simulink model "TFlex_PID"  (R2018a)
settings: Solver=FixedStepDiscrete  StartTime=0.0  StopTime=t_end  FixedStep=ts  RelTol=1e-3
PreLoadFcn:
  | Ts = 0.001;
InitFcn:
  | Ts = 0.001;
values from neighbouring files (symbols this model uses):
  a0 = omega_n^3    (= 31006276.6803)    [Tflex_PID_init.m]
  a1 = 3*omega_n^2    (= 296088.132033)    [Tflex_PID_init.m]
  a2 = 3*omega_n    (= 942.477796077)    [Tflex_PID_init.m]
  b = ones(2*D,Q)*0.001    [Tflex_PID_init.m]
  D = 21    [Tflex_PID_init.m]
  I_limit_max = 500    [Tflex_PID_init.m]
  I_limit_min = -500    [Tflex_PID_init.m]
  Kd = kp*(tau_z-tau_p*(1+(tau_z+tau_p)/tau_i))    [Tflex_PID_init.m]
  Ki = kp/tau_i    [Tflex_PID_init.m]
  Kp = kp*(1+(tau_z-tau_p)/tau_i)    [Tflex_PID_init.m]
  kp = m_eq*crossOver^2/sqrt(1/alpha)    [Tflex_PID_init.m]
  R = eye(2*D,2*D)*sn^2    [Tflex_PID_init.m]
  sf = 185.90    (= 185.9)    [Tflex_PID_init.m]
  t_end = 200    [Tflex_PID_init.m]    (also in multisineInit.m = t(end))
  tau_i = beta*tau_z    [Tflex_PID_init.m]
  tau_p = 1/(crossOver*sqrt(1/alpha))    [Tflex_PID_init.m]
  tau_z = sqrt(1/alpha)/crossOver    [Tflex_PID_init.m]
  ts = 1/1000    (= 0.001)    [Tflex_PID_init.m]    (also in init.m = 0.00025; multisineInit.m)
  w = ones(2*D,Q)*0.001    [Tflex_PID_init.m]
undefined symbols (not defined in the file or in its folder): DiscIntNeverNeededParam, LPden, LPnum, SIGMA
libraries: xpcethercatlib x91, simulink x61, slrtlib x9
(part 1 of 2)
settings Model: xpc_rtwmakecfg_data=_xpcethercatlib_  SimulationMode=external  ExtModeTrigDirection=either  ExplicitPartitioning=on  Creator=lab  LastModifiedBy=wout7
settings SolverCC: AutoInsertRateTranBlk=on
settings DataIOCC: Decimation=10  LimitDataPoints=on  SaveFormat=StructureWithTime
settings OptimizationCC: BlockReduction=off  OptimizeBlockIOStorage=off  BufferReuse=off  GlobalBufferReuse=off  ExpressionFolding=off  LocalBlockOutputs=off  OptimizeDataStoreBuffers=off  BusAssignmentInplaceUpdate=off
settings DebuggingCC: UnconnectedInputMsg=none  UnconnectedOutputMsg=none  UnconnectedLineMsg=none
settings HardwareCC: ProdBitPerPointer=32  ProdBitPerSizeT=32  ProdBitPerPtrDiffT=32  ProdLargestAtomicFloat=None  ProdWordSize=32  ProdLongLongMode=on  ProdHWDeviceType=Generic->32-bit x86 compatible
settings RTWCC: SystemTargetFile=slrt.tlc  TemplateMakefile=slrt_default_tmf  Description=Simulink Real-Time  CodeExecutionProfiling=on
settings SimulinkRealTimeCC: SupportVariableSizeSignals=on  xPCConcurrentTasks=on

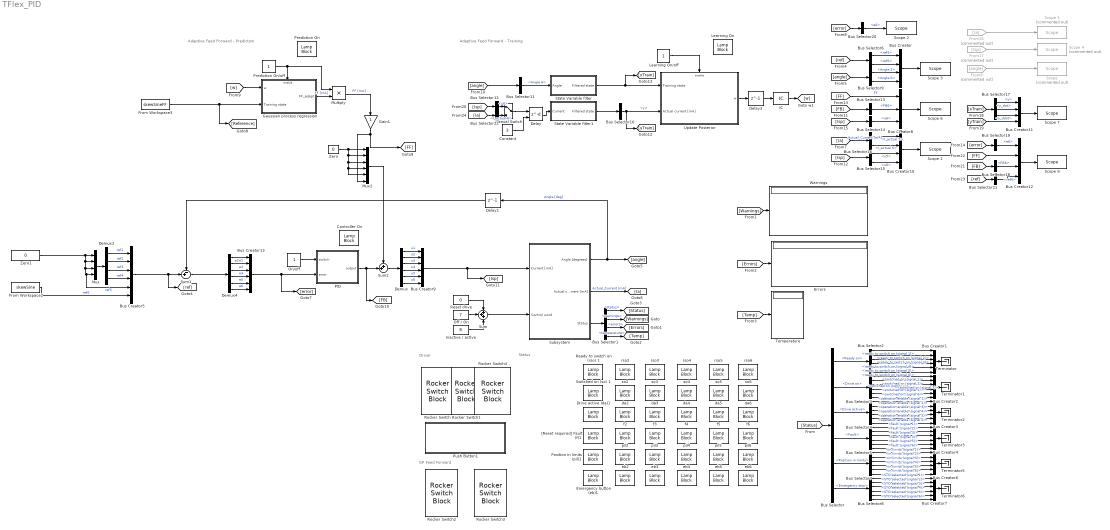
== system TFlex_PID ==
  note: GP Feed Forward
  note: Driver
  note: Status
  note: Adaptive Feed Forward - Prediction
  note: Adaptive Feed Forward - Training
  " da2 " : LampBlock  WebBlockId=1372  LabelPosition=Hide
  " so2 " : LampBlock  WebBlockId=1336  LabelPosition=Hide
  " da4" : LampBlock  WebBlockId=1373  LabelPosition=Hide
  " da5" : LampBlock  WebBlockId=1374  LabelPosition=Hide
  " da6" : LampBlock  WebBlockId=1375  LabelPosition=Hide
  " eb4" : LampBlock  WebBlockId=1402  LabelPosition=Hide
  " eb5" : LampBlock  WebBlockId=1403  LabelPosition=Hide
  " eb6" : LampBlock  WebBlockId=1404  LabelPosition=Hide
  " f4" : LampBlock  WebBlockId=1379  LabelPosition=Hide
  " f5" : LampBlock  WebBlockId=1380  LabelPosition=Hide
  " f6" : LampBlock  WebBlockId=1381  LabelPosition=Hide
  " pil4" : LampBlock  WebBlockId=1397  LabelPosition=Hide
  " pil5" : LampBlock  WebBlockId=1398  LabelPosition=Hide
  " pil6" : LampBlock  WebBlockId=1399  LabelPosition=Hide
  " rso4" : LampBlock  WebBlockId=1325  LabelPosition=Hide
  " so4" : LampBlock  WebBlockId=1333  LabelPosition=Hide
  " so5" : LampBlock  WebBlockId=1334  LabelPosition=Hide
  " so6" : LampBlock  WebBlockId=1335  LabelPosition=Hide
  Bus Creator{,10..12} (4 alike) : BusCreator  Inputs=4
  Bus Creator{1..7,9,13} (9 alike) : BusCreator  Inputs=6
  Bus Creator8 : BusCreator  Inputs=3
  Bus Selector : BusSelector  OutputSignals=Ready on,Drive on,Drive active,Fault,Position in limits,Emergency stop
  Bus Selector1 : BusSelector  OutputSignals=status,warnings,errors,temperature
  Bus Selector10 : BusSelector  OutputSignals=y
  Bus Selector11 : BusSelector  OutputSignals=Angle 6
  Bus Selector12 : BusSelector  OutputSignals=u6
  Bus Selector13 : BusSelector  OutputSignals=FB6
  Bus Selector14 : BusSelector  OutputSignals=u6
  Bus Selector15 : BusSelector  OutputSignals=u5,u6
  Bus Selector16 : BusSelector  OutputSignals=I_actual 5,I_actual 6
  Bus Selector17 : BusSelector  OutputSignals=y,y_dot,y_ddot
  Bus Selector18 : BusSelector  OutputSignals=FB6
  Bus Selector19 : BusSelector  OutputSignals=e6
  Bus Selector2 : BusSelector  OutputSignals=ready to switch on (signal 1),ready to switch on (signal 2),ready to switch on (signal 3),ready to switch on (signal 4),ready to switch on (signal 5),ready to switch on (signal 6)
  Bus Selector20 : BusSelector  OutputSignals=e6
  Bus Selector21 : BusSelector  OutputSignals=ref6
  Bus Selector22 : BusSelector  OutputSignals=I_actual 6
  Bus Selector3 : BusSelector  OutputSignals=switched on (signal 1),switched on (signal 2),switched on (signal 3),switched on (signal 4),switched on (signal 5),switched on (signal 6)
  Bus Selector4 : BusSelector  OutputSignals=operation enable (signal 1),operation enable (signal 2),operation enable (signal 3),operation enable (signal 4),operation enable (signal 5),operation enable (signal 6)
  Bus Selector5 : BusSelector  OutputSignals=fault (signal 1),fault (signal 2),fault (signal 3),fault (signal 4),fault (signal 5),fault (signal 6)
  Bus Selector6 : BusSelector  OutputSignals=ref5,ref6
  Bus Selector7 : BusSelector  OutputSignals=in limits (signal 1),in limits (signal 2),in limits (signal 3),in limits (signal 4),in limits (signal 5),in limits (signal 6)
  Bus Selector8 : BusSelector  OutputSignals=STO selected (signal 1),STO selected (signal 2),STO selected (signal 3),STO selected (signal 4),STO selected (signal 5),STO selected (signal 6)
  Bus Selector9 : BusSelector  OutputSignals=Angle 5,Angle 6
  Constant : Constant  Value=3  SampleTime=ts
  "Controller On " : LampBlock  WebBlockId=1976  LabelPosition=Hide
  Delay : Delay  DelayLengthSource=Input port
      settings: InputPortMap=u0,p1
  Delay1 : Delay  DelayLength=1
  Delay3 : Delay  DelayLength=1  InitialCondition=0
  Demux : Demux  Outputs=6
  Demux2 : Demux
  Demux4 : Demux  Outputs=6
  Drive active (da)1 : LampBlock  WebBlockId=1376
  Emergency button (eb)1 : LampBlock  WebBlockId=1405
  Errors : Display
      settings: Decimation=25
  From Workspace2 : FromWorkspace  VariableName=skewSine  SampleTime=ts  OutputAfterFinalValue=Setting to zero
  From Workspace3 : FromWorkspace  VariableName=skewSineFF  SampleTime=ts  OutputAfterFinalValue=Setting to zero
  From16 : From  Commented=on  GotoTag=Ia
  From17 : From  Commented=on  GotoTag=Isp
  From6 : From  Commented=on  GotoTag=angle
  Gain1 : Gain
  Gaussian process regression : Subsystem
  IC : InitialCondition  Value=w
  Inactive / active : Constant  Value=8  SampleTime=-1
  Learning On : LampBlock  WebBlockId=2313  LabelPosition=Hide
  Learning On/off : Constant  SampleTime=ts
  Manual Switch : ManualSwitch
  Multiply : Product
  Mux : Mux
  Mux2 : Mux  Inputs=6
  Off / On : Constant  Value=7  SampleTime=-1
  On/off : Constant  SampleTime=ts
  "PID " : Subsystem
  Position in limits (pil)1 : LampBlock  WebBlockId=1400
  "Prediction On " : LampBlock  WebBlockId=2312  LabelPosition=Hide
  Prediction On/off : Constant  SampleTime=ts
  Push Button1 : Subsystem  DialogController=hmiCreateDDGDialog  IsWebBlock=on  mask(MWDashboardBlock){webBlockId=c834c18b-4d14-4fd2-a2aa-8470ccae1b8a, webBlockType=pushbutton, ShowInLibBrwoser=on, ShowInitialText=on, HMISrcModelName=TFlex_PID}
      mask prompts: webBlockId "WebBlock Id"; webBlockType "WebBlock Type"; HMISrcModelName "Source Model"
      mask help: SimulinkHMI:dialogs:PushButtonDialogDesc
      mask Help: helpview([docroot '/mapfiles/simulink.map'], 'hmi_push_button')
      mask Display:
      | model = bdroot(gcb);
      | if strcmp(get_param(model,'BlockDiagramType'), 'library')
      |     image([(matlabroot) '/toolbox/simulink/hmi/icons/PushButton.png']);
      | end
  Ready to switch on (rso) 1 : LampBlock  WebBlockId=226
  Reset drive : Constant  Value=0  SampleTime=-1
  Rocker Switch : RockerSwitchBlock  WebBlockId=231  LabelPosition=Hide
      settings: Values={{'Off', 'Driver On'}, [6 7]}
  Rocker Switch1 : RockerSwitchBlock  WebBlockId=232  LabelPosition=Hide
      settings: Values={{'Off', 'Driver Active'}, [0 8]}
  Rocker Switch2 : RockerSwitchBlock  WebBlockId=2309  LabelPosition=Hide
      settings: Values={{'Off', 'Prediction On'}, [0 1]}
  Rocker Switch3 : RockerSwitchBlock  WebBlockId=2310  LabelPosition=Hide
      settings: Values={{'Off', 'Learning On'}, [0 1]}
  Rocker Switch4 : RockerSwitchBlock  WebBlockId=1973  LabelPosition=Hide
      settings: Values={{'Off', 'Controller On'}, [0 1]}
  "Scope " : slrtlib/Displays and Logging/Scope   Commented=on  scopeno=1  scopetype=File  autostart=on  viewmode=Graphical redraw  formatstr='%15.6f'  grid=on  ylimits=[0,0]  nosamples=t_end/ts  noprepostsamples=0  interleave=1  triggermode=FreeRun  triggersignal=1  trigsignalfromport=off  triggerlevel=0.0  triggerslope=Either  triggerscope=1  triggersample=0  filename=ANGLE.dat  mode=Lazy  writesize=512  autorestart=off  dynamicfilemode=off  maxwritefilesize=512*1024^2
  Scope 1 : slrtlib/Displays and Logging/Scope   scopeno=2  scopetype=Target  autostart=on  viewmode=Graphical sliding  formatstr='%15.6f,%15.6f,%15.6f,%15.6f,%15.6f,%15.6f'  grid=on  ylimits=[-500 500]  nosamples=2000  noprepostsamples=0  interleave=25  triggermode=FreeRun  triggersignal=1  trigsignalfromport=off  triggerlevel=0.0  triggerslope=Either  triggerscope=1  triggersample=0  filename=data.dat  mode=Lazy  writesize=512  autorestart=off  dynamicfilemode=off  maxwritefilesize=512*1024^2
  Scope 2 : slrtlib/Displays and Logging/Scope   scopeno=4  scopetype=Target  autostart=on  viewmode=Graphical sliding  formatstr='%15.6f,%15.6f,%15.6f,%15.6f,%15.6f,%15.6f'  grid=on  ylimits=[-1e-1 1e-1]  nosamples=2000  noprepostsamples=0  interleave=25  triggermode=FreeRun  triggersignal=1  trigsignalfromport=off  triggerlevel=0.0  triggerslope=Either  triggerscope=1  triggersample=0  filename=data.dat  mode=Lazy  writesize=512  autorestart=off  dynamicfilemode=off  maxwritefilesize=512*1024^2
  Scope 3 : slrtlib/Displays and Logging/Scope   scopeno=3  scopetype=Target  autostart=on  viewmode=Graphical sliding  formatstr='%15.6f,%15.6f,%15.6f,%15.6f,%15.6f,%15.6f'  grid=on  ylimits=[-30,30]  nosamples=2000  noprepostsamples=0  interleave=25  triggermode=FreeRun  triggersignal=1  trigsignalfromport=off  triggerlevel=0.0  triggerslope=Either  triggerscope=1  triggersample=0  filename=data.dat  mode=Lazy  writesize=512  autorestart=off  dynamicfilemode=off  maxwritefilesize=512*1024^2
  Scope 4 : slrtlib/Displays and Logging/Scope   Commented=on  scopeno=5  scopetype=File  autostart=on  viewmode=Graphical redraw  formatstr='%15.6f'  grid=on  ylimits=[0,0]  nosamples=t_end/ts  noprepostsamples=0  interleave=1  triggermode=FreeRun  triggersignal=1  trigsignalfromport=off  triggerlevel=0.0  triggerslope=Either  triggerscope=1  triggersample=0  filename=I_SP.dat  mode=Lazy  writesize=512  autorestart=off  dynamicfilemode=off  maxwritefilesize=512*1024^2
  Scope 5 : slrtlib/Displays and Logging/Scope   Commented=on  scopeno=6  scopetype=File  autostart=on  viewmode=Graphical redraw  formatstr='%15.6f'  grid=on  ylimits=[0,0]  nosamples=t_end/ts  noprepostsamples=0  interleave=1  triggermode=FreeRun  triggersignal=1  trigsignalfromport=off  triggerlevel=0.0  triggerslope=Either  triggerscope=1  triggersample=0  filename=I_A.dat  mode=Lazy  writesize=512  autorestart=off  dynamicfilemode=off  maxwritefilesize=512*1024^2
  Scope 6 : slrtlib/Displays and Logging/Scope   scopeno=7  scopetype=Target  autostart=on  viewmode=Graphical sliding  formatstr='%15.6f,%15.6f,%15.6f,%15.6f,%15.6f,%15.6f'  grid=on  ylimits=[-500 500]  nosamples=2000  noprepostsamples=0  interleave=25  triggermode=FreeRun  triggersignal=1  trigsignalfromport=off  triggerlevel=0.0  triggerslope=Either  triggerscope=1  triggersample=0  filename=data.dat  mode=Lazy  writesize=512  autorestart=off  dynamicfilemode=off  maxwritefilesize=512*1024^2
  Scope 7 : slrtlib/Displays and Logging/Scope   scopeno=8  scopetype=File  autostart=on  viewmode=Graphical redraw  formatstr='%15.6f'  grid=on  ylimits=[0,0]  nosamples=t_end/ts  noprepostsamples=0  interleave=1  triggermode=FreeRun  triggersignal=1  trigsignalfromport=off  triggerlevel=0.0  triggerslope=Either  triggerscope=1  triggersample=0  filename=TRAIN.dat  mode=Lazy  writesize=512  autorestart=off  dynamicfilemode=off  maxwritefilesize=512*1024^2
  Scope 9 : slrtlib/Displays and Logging/Scope   scopeno=10  scopetype=File  autostart=on  viewmode=Graphical redraw  formatstr='%15.6f'  grid=on  ylimits=[0,0]  nosamples=t_end/ts  noprepostsamples=0  interleave=1  triggermode=FreeRun  triggersignal=1  trigsignalfromport=off  triggerlevel=0.0  triggerslope=Either  triggerscope=1  triggersample=0  filename=Error.dat  mode=Lazy  writesize=512  autorestart=off  dynamicfilemode=off  maxwritefilesize=512*1024^2
  State Variable filter : Subsystem
  State Variable filter1 : Subsystem
  Subsystem : Subsystem  TreatAsAtomicUnit=on
  Sum : Sum  Inputs=+++
  Sum1 : Sum  Inputs=-+|
  Sum2 : Sum  Inputs=++|
  Switched on (so) 1 : LampBlock  WebBlockId=1338
  Temperature : Display
      settings: Decimation=25
  Terminator{,1..3,5..6} (6 alike) : Terminator
  Update Posterior : Subsystem
  Warnings : Display
      settings: Decimation=25
  Zero : Constant  Value=0
  Zero1 : Constant  Value=0  SampleTime=ts
  "[Reset required] Fault (f)1 " : LampBlock  WebBlockId=1382
  da3 : LampBlock  WebBlockId=1377  LabelPosition=Hide
  eb2 : LampBlock  WebBlockId=1406  LabelPosition=Hide
  eb3 : LampBlock  WebBlockId=1407  LabelPosition=Hide
  f2 : LampBlock  WebBlockId=1378  LabelPosition=Hide
  f3 : LampBlock  WebBlockId=1383  LabelPosition=Hide
  pil2 : LampBlock  WebBlockId=1396  LabelPosition=Hide
  pil3 : LampBlock  WebBlockId=1401  LabelPosition=Hide
  rso2 : LampBlock  WebBlockId=1323  LabelPosition=Hide
  rso3 : LampBlock  WebBlockId=1324  LabelPosition=Hide
  rso5 : LampBlock  WebBlockId=1326  LabelPosition=Hide
  rso6 : LampBlock  WebBlockId=1327  LabelPosition=Hide
  so3 : LampBlock  WebBlockId=1337  LabelPosition=Hide
  wires:
  [Ia] -> Bus Selector16/1  "Actual_Current [mA]"
  Bus Selector/1 -> Bus Selector2/1  "<Ready on>"
  Bus Selector/2 -> Bus Selector3/1  "<Drive on>"
  Bus Selector/3 -> Bus Selector4/1  "<Drive active>"
  Bus Selector/4 -> Bus Selector5/1  "<Fault>"
  Bus Selector/5 -> Bus Selector7/1  "<Position in limits>"
  Bus Selector/6 -> Bus Selector8/1  "<Emergency stop>"
  Reset drive/1 -> Sum/1
  Off / On/1 -> Sum/2
  Inactive / active/1 -> Sum/3
  Subsystem/1(Angle [degrees]) -> Delay1/1, [angle]  "Angle [deg]"
  Subsystem/3(Status) -> Bus Selector1/1
  [Temp] -> Temperature/1
  [Errors] -> Errors/1
  [Warnings] -> Warnings/1
  [Status] -> Bus Selector/1
  Bus Selector2/1 -> Bus Creator1/1  "<ready to switch on (signal 1)>"
  Bus Selector2/2 -> Bus Creator1/2  "<ready to switch on (signal 2)>"
  Bus Selector2/3 -> Bus Creator1/3  "<ready to switch on (signal 3)>"
  Bus Selector2/4 -> Bus Creator1/4  "<ready to switch on (signal 4)>"
  Bus Selector2/5 -> Bus Creator1/5  "<ready to switch on (signal 5)>"
  Bus Selector2/6 -> Bus Creator1/6  "<ready to switch on (signal 6)>"
  Bus Creator1/1 -> Terminator/1
  Bus Selector3/2 -> Bus Creator2/2  "<switched on (signal 2)>"
  Bus Selector3/1 -> Bus Creator2/1  "<switched on (signal 1)>"
  Bus Selector3/5 -> Bus Creator2/5  "<switched on (signal 5)>"
  Bus Creator2/1 -> Terminator1/1
  Bus Selector3/4 -> Bus Creator2/4  "<switched on (signal 4)>"
  Bus Selector3/6 -> Bus Creator2/6  "<switched on (signal 6)>"
  Bus Selector3/3 -> Bus Creator2/3  "<switched on (signal 3)>"
  Bus Selector4/4 -> Bus Creator3/4  "<operation enable (signal 4)>"
  Bus Selector4/6 -> Bus Creator3/6  "<operation enable (signal 6)>"
  Bus Creator3/1 -> Terminator2/1
  Bus Selector4/5 -> Bus Creator3/5  "<operation enable (signal 5)>"
  Bus Selector4/1 -> Bus Creator3/1  "<operation enable (signal 1)>"
  Bus Selector4/2 -> Bus Creator3/2  "<operation enable (signal 2)>"
  Bus Selector4/3 -> Bus Creator3/3  "<operation enable (signal 3)>"
  Bus Selector5/4 -> Bus Creator4/4  "<fault (signal 4)>"
  Bus Selector5/6 -> Bus Creator4/6  "<fault (signal 6)>"
  Bus Creator4/1 -> Terminator3/1
  Bus Selector5/5 -> Bus Creator4/5  "<fault (signal 5)>"
  Bus Selector5/1 -> Bus Creator4/1  "<fault (signal 1)>"
  Bus Selector5/2 -> Bus Creator4/2  "<fault (signal 2)>"
  Bus Selector5/3 -> Bus Creator4/3  "<fault (signal 3)>"
  Bus Selector7/4 -> Bus Creator6/4  "<in limits (signal 4)>"
  Bus Selector7/6 -> Bus Creator6/6  "<in limits (signal 6)>"
  Bus Creator6/1 -> Terminator5/1
  Bus Selector7/5 -> Bus Creator6/5  "<in limits (signal 5)>"
  Bus Selector7/1 -> Bus Creator6/1  "<in limits (signal 1)>"
  Bus Selector7/2 -> Bus Creator6/2  "<in limits (signal 2)>"
  Bus Selector7/3 -> Bus Creator6/3  "<in limits (signal 3)>"
  Bus Selector8/4 -> Bus Creator7/4  "<STO selected (signal 4)>"
  Bus Selector8/6 -> Bus Creator7/6  "<STO selected (signal 6)>"
  Bus Creator7/1 -> Terminator6/1
  Bus Selector8/5 -> Bus Creator7/5  "<STO selected (signal 5)>"
  Bus Selector8/1 -> Bus Creator7/1  "<STO selected (signal 1)>"
  Bus Selector8/2 -> Bus Creator7/2  "<STO selected (signal 2)>"
  Bus Selector8/3 -> Bus Creator7/3  "<STO selected (signal 3)>"
  Bus Creator9/1 -> [Isp], Subsystem/1(Current [mA])
  Sum/1 -> Subsystem/2(Control word)
  Bus Selector1/1 -> [Status]  "<status>"
  Bus Selector1/2 -> [Warnings]  "<warnings>"
  Bus Selector1/3 -> [Errors]  "<errors>"
  Bus Selector1/4 -> [Temp]  "<temperature>"
  Bus Creator13/1 -> [error], "PID "/2(error)
  On/off/1 -> "PID "/1(switch)
  Zero1/1 -> Bus Creator5/5, Mux/4, Mux/3, Mux/2, Mux/1  "ref5"
  Demux2/3 -> Bus Creator5/3  "ref3"
  Bus Creator5/1 -> [ref], Sum1/2
  Demux2/4 -> Bus Creator5/4  "ref4"
  Demux2/2 -> Bus Creator5/2  "ref2"
  Mux/1 -> Demux2/1
  Demux2/1 -> Bus Creator5/1  "ref1"
  [ref] -> Bus Selector6/1
  [angle] -> Bus Selector9/1
  Bus Selector6/1 -> Bus Creator/1  "<ref5>"
  Bus Selector6/2 -> Bus Creator/2  "<ref6>"
  Bus Selector9/1 -> Bus Creator/3  "<Angle 5>"
  Bus Selector9/2 -> Bus Creator/4  "<Angle 6>"
  Bus Creator/1 -> Scope 3/1
  Subsystem/2(Actual current [mA]) -> [Ia]  "Actual_Current [mA]"
  From6/1 -> "Scope "/1
  State Variable filter1/1(Filtered state) -> Bus Selector10/1
  Delay3/1 -> IC/1
  [Isp] -> Bus Selector12/1
  Bus Selector11/1 -> State Variable filter/1(Angle)  "<Angle 6>"
  Bus Selector10/1 -> Update Posterior/2("Actual current [mA] "), [yTrain]  "<y>"
  Multiply/1 -> Gain1/1  "FF [mA]"
  From Workspace3/1 -> Gaussian process regression/2(Training state), [Reference]
  Gaussian process regression/1(FF_adapt) -> Multiply/2  "FF [mA]"
  Learning On/off/1 -> Update Posterior/Enable
  Update Posterior/1(w) -> Delay3/1
  [w] -> Gaussian process regression/1(w)
  IC/1 -> [w]
  Prediction On/off/1 -> Gaussian process regression/Enable, Multiply/1
  [Isp] -> Bus Selector15/1
  [angle] -> Bus Selector11/1
  [FB] -> Bus Selector13/1
  [Isp] -> Bus Selector14/1
  [FF] -> Bus Creator8/1  "FF"
  Bus Creator8/1 -> Scope 6/1
  "PID "/1(output) -> [FB], Sum2/2
  Mux2/1 -> Sum2/1
  Sum2/1 -> Demux/1
  Demux/6 -> Bus Creator9/6  "u6"
  Demux/5 -> Bus Creator9/5  "u5"
  Demux/4 -> Bus Creator9/4  "u4"
  Demux/3 -> Bus Creator9/3  "u3"
  Demux/2 -> Bus Creator9/2  "u2"
  Demux/1 -> Bus Creator9/1  "u1"
  From Workspace2/1 -> Bus Creator5/6  "ref6"
  Bus Selector16/1 -> Bus Creator10/1  "<I_actual 5>"
  Bus Selector16/2 -> Bus Creator10/2  "<I_actual 6>"
  Bus Selector15/1 -> Bus Creator10/3  "<u5>"
  Bus Selector15/2 -> Bus Creator10/4  "<u6>"
  Bus Selector13/1 -> Bus Creator8/2  "<FB6>"
  Bus Selector14/1 -> Bus Creator8/3  "<u6>"
  Bus Creator10/1 -> Scope 1/1
  From16/1 -> Scope 5/1
  From17/1 -> Scope 4/1
  State Variable filter/1(Filtered state) -> [xTrain], Update Posterior/1(Training state)
  [xTrain] -> Bus Selector17/1
  Bus Selector17/1 -> Bus Creator11/1  "<y>"
  Bus Selector17/2 -> Bus Creator11/2  "<y_dot>"
  Bus Selector17/3 -> Bus Creator11/3  "<y_ddot>"
  [yTrain] -> Bus Creator11/4
  Bus Creator11/1 -> Scope 7/1
  Gain1/1 -> Mux2/6, [FF]
  Zero/1 -> Mux2/5, Mux2/4, Mux2/3, Mux2/2, Mux2/1
  Manual Switch/1 -> Delay/1
  Delay/1 -> State Variable filter1/1(Current)
  [error] -> Bus Selector19/1
  [FB] -> Bus Selector18/1
  Bus Selector18/1 -> Bus Creator12/3  "<FB6>"
  [FF] -> Bus Creator12/2
  Bus Creator12/1 -> Scope 9/1
  Demux4/6 -> Bus Creator13/6  "e6"
  Demux4/5 -> Bus Creator13/5  "e5"
  Demux4/1 -> Bus Creator13/1  "e1"
  Demux4/3 -> Bus Creator13/3  "e3"
  Demux4/2 -> Bus Creator13/2  "e2"
  Demux4/4 -> Bus Creator13/4  "e4"
  Bus Selector19/1 -> Bus Creator12/1  "<e6>"
  [error] -> Bus Selector20/1
  Bus Selector20/1 -> Scope 2/1  "<e6>"
  Sum1/1 -> Demux4/1
  Delay1/1 -> Sum1/1
  [ref] -> Bus Selector21/1
  Bus Selector21/1 -> Bus Creator12/4  "<ref6>"
  [Ia] -> Bus Selector22/1
  Constant/1 -> Delay/2
  Bus Selector12/1 -> Manual Switch/1  "<u6>"
  Bus Selector22/1 -> Manual Switch/2  "<I_actual 6>"

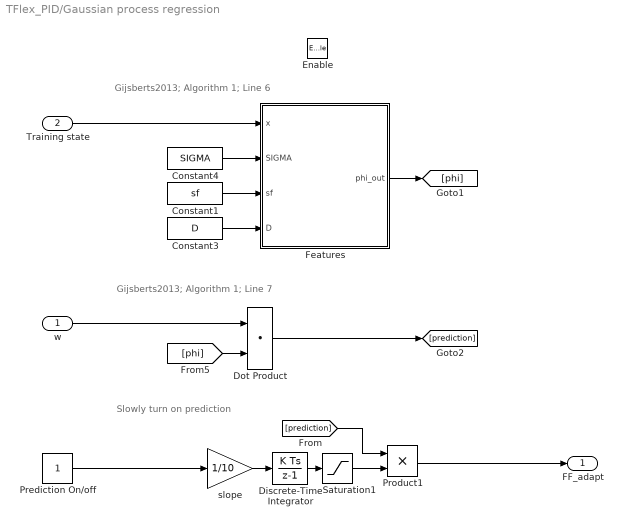
== system TFlex_PID/Gaussian process regression ==
  note: Gijsberts2013; Algorithm 1; Line 7
  note: Gijsberts2013; Algorithm 1; Line 6
  note: Slowly turn on prediction
  w : Inport
  Training state : Inport  Port=2
  Enable : EnablePort  StatesWhenEnabling=reset
  Constant1 : Constant  Value=sf  VectorParams1D=off
  Constant3 : Constant  Value=D  VectorParams1D=off
  Constant4 : Constant  Value=SIGMA  VectorParams1D=off
  Discrete-Time Integrator : DiscreteIntegrator  SampleTime=-1  ICPrevOutput=DiscIntNeverNeededParam  ICPrevScaledInput=DiscIntNeverNeededParam
  Dot Product : DotProduct  OutDataTypeStr=Inherit: Inherit via internal rule
  Features : Subsystem
  Prediction On/off : Constant
  Product1 : Product
  Saturation1 : Saturate  UpperLimit=1  LowerLimit=0
  slope : Gain  Gain=1/10
  FF_adapt : Outport  SampleTime=ts
  wires:
  w/1 -> Dot Product/1
  [phi] -> Dot Product/2
  Product1/1 -> FF_adapt/1
  slope/1 -> Discrete-Time Integrator/1
  Prediction On/off/1 -> slope/1
  Discrete-Time Integrator/1 -> Saturation1/1
  Dot Product/1 -> [prediction]
  Constant4/1 -> Features/2(SIGMA)
  Training state/1 -> Features/1(x)
  Features/1(phi_out) -> [phi]
  Constant3/1 -> Features/4(D)
  Constant1/1 -> Features/3(sf)
  Saturation1/1 -> Product1/2
  [prediction] -> Product1/1

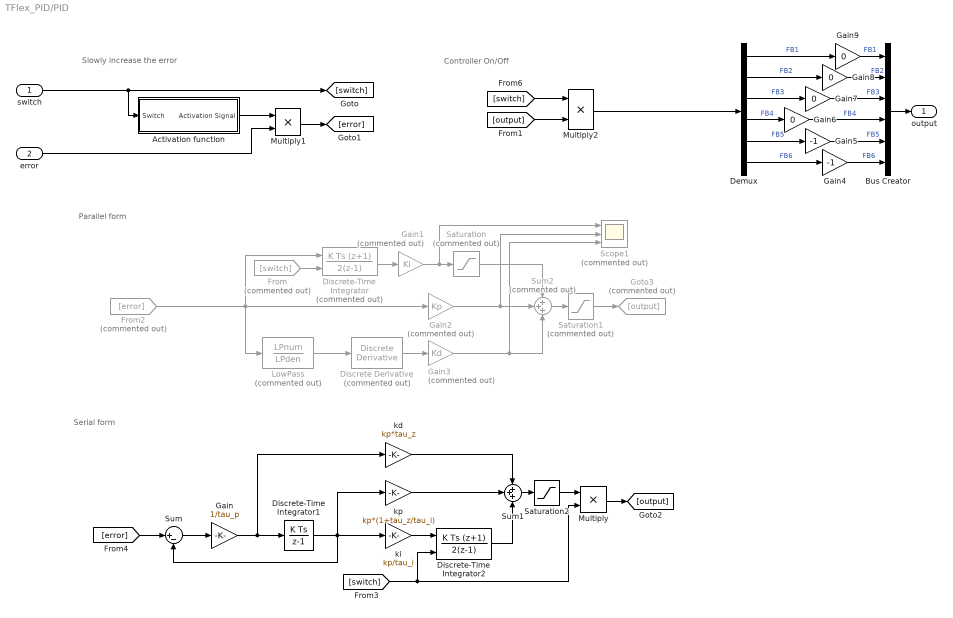
== system TFlex_PID/PID  ==
  note: Controller On/Off
  note: Slowly increase the error
  note: Serial form
  note: Parallel form
  switch : Inport  SampleTime=ts
  error : Inport  Port=2
  Activation function : Subsystem
  Bus Creator : BusCreator  Inputs=6
  Demux : Demux  Outputs=6
  Discrete Derivative : simulink/Discrete/Discrete Derivative  Commented=on  gainval=1.0  ICPrevScaledInput=0.0  OutMin=[]  OutMax=[]  OutDataType=fixdt(1, 16)  OutScaling=2^-10  DoSatur=off
  Discrete-Time Integrator : DiscreteIntegrator  Commented=on  IntegratorMethod=Integration: Trapezoidal  ExternalReset=either  SampleTime=ts  LimitOutput=on  UpperSaturationLimit=I_limit_max  LowerSaturationLimit=I_limit_min  ICPrevOutput=DiscIntNeverNeededParam  ICPrevScaledInput=DiscIntNeverNeededParam
  Discrete-Time Integrator1 : DiscreteIntegrator  SampleTime=-1  ICPrevOutput=DiscIntNeverNeededParam  ICPrevScaledInput=DiscIntNeverNeededParam
  Discrete-Time Integrator2 : DiscreteIntegrator  IntegratorMethod=Integration: Trapezoidal  ExternalReset=rising  SampleTime=ts  LimitOutput=on  UpperSaturationLimit=I_limit_max  LowerSaturationLimit=I_limit_min  ICPrevOutput=DiscIntNeverNeededParam  ICPrevScaledInput=DiscIntNeverNeededParam
  From : From  Commented=on  GotoTag=switch
  From2 : From  Commented=on  GotoTag=error
  Gain : Gain  Gain=1/tau_p
  Gain1 : Gain  Commented=on  Gain=Ki
  Gain2 : Gain  Commented=on  Gain=Kp
  Gain3 : Gain  Commented=on  Gain=Kd
  Gain4 : Gain  Gain=-1
  Gain5 : Gain  Gain=-1
  Gain{6..9} (4 alike) : Gain  Gain=0
  Goto3 : Goto  Commented=on  GotoTag=output
  LowPass : DiscreteTransferFcn  Commented=on  Numerator=LPnum  Denominator=LPden
  Multiply : Product
  Multiply1 : Product
  Multiply2 : Product
  Saturation : Saturate  Commented=on  UpperLimit=I_limit_max  LowerLimit=I_limit_min
  Saturation1 : Saturate  Commented=on  UpperLimit=I_limit_max  LowerLimit=I_limit_min
  Saturation2 : Saturate  UpperLimit=I_limit_max  LowerLimit=I_limit_min
  Scope1 : Scope  Commented=on  NumInputPorts=3
  Sum : Sum  Inputs=|+-
  Sum1 : Sum  Inputs=+++
  Sum2 : Sum  Commented=on  Inputs=+++
  kd : Gain  Gain=kp*tau_z
  ki : Gain  Gain=kp/tau_i
  kp : Gain  Gain=kp*(1+tau_z/tau_i)
  output : Outport
  wires:
  LowPass/1 -> Discrete Derivative/1
  From2/1 -> Discrete-Time Integrator/1, Gain2/1, LowPass/1
  Discrete-Time Integrator/1 -> Gain1/1
  Gain2/1 -> Scope1/2, Sum2/2
  Gain3/1 -> Scope1/3, Sum2/3
  Sum2/1 -> Saturation1/1
  Sum/1 -> Gain/1
  Gain/1 -> Discrete-Time Integrator1/1, kd/1
  ki/1 -> Discrete-Time Integrator2/1
  Discrete-Time Integrator1/1 -> kp/1, ki/1, Sum/2
  kp/1 -> Sum1/2
  kd/1 -> Sum1/1
  Discrete-Time Integrator2/1 -> Sum1/3
  Discrete Derivative/1 -> Gain3/1
  [error] -> Sum/1
  Sum1/1 -> Saturation2/1
  [switch] -> Discrete-Time Integrator2/2, Multiply/2
  Multiply/1 -> [output]
  switch/1 -> [switch], Activation function/1(Switch)
  error/1 -> Multiply1/2
  [output] -> Multiply2/2
  From/1 -> Discrete-Time Integrator/2
  Multiply1/1 -> [error]
  [switch] -> Multiply2/1
  Bus Creator/1 -> output/1
  Gain1/1 -> Saturation/1, Scope1/1
  Activation function/1(Activation Signal) -> Multiply1/1
  Saturation1/1 -> Goto3/1
  Multiply2/1 -> Demux/1
  Gain4/1 -> Bus Creator/6  "FB6"
  Demux/6 -> Gain4/1  "FB6"
  Demux/5 -> Gain5/1  "FB5"
  Demux/4 -> Gain6/1  "FB4"
  Demux/3 -> Gain7/1  "FB3"
  Demux/1 -> Gain9/1  "FB1"
  Demux/2 -> Gain8/1  "FB2"
  Gain5/1 -> Bus Creator/5  "FB5"
  Gain6/1 -> Bus Creator/4  "FB4"
  Gain7/1 -> Bus Creator/3  "FB3"
  Gain8/1 -> Bus Creator/2  "FB2"
  Gain9/1 -> Bus Creator/1  "FB1"
  Saturation/1 -> Sum2/1
  Saturation2/1 -> Multiply/1

== system TFlex_PID/Push Button1 ==

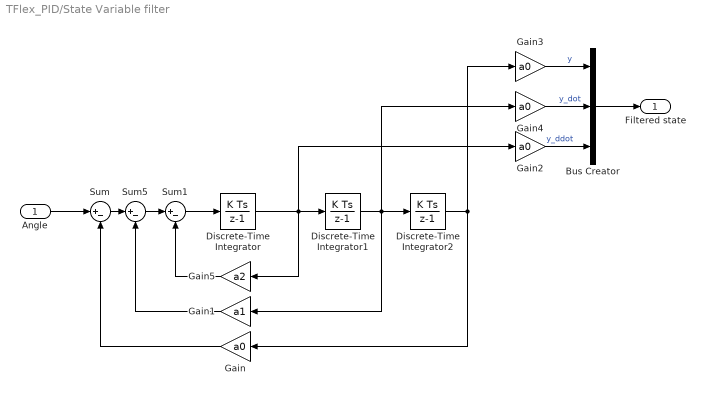
== system TFlex_PID/State Variable filter ==
  Angle : Inport
  Bus Creator : BusCreator  Inputs=3
  Discrete-Time Integrator : DiscreteIntegrator  SampleTime=-1  ICPrevOutput=DiscIntNeverNeededParam  ICPrevScaledInput=DiscIntNeverNeededParam
  Discrete-Time Integrator1 : DiscreteIntegrator  SampleTime=-1  ICPrevOutput=DiscIntNeverNeededParam  ICPrevScaledInput=DiscIntNeverNeededParam
  Discrete-Time Integrator2 : DiscreteIntegrator  SampleTime=-1  ICPrevOutput=DiscIntNeverNeededParam  ICPrevScaledInput=DiscIntNeverNeededParam
  Gain{,2..4} (4 alike) : Gain  Gain=a0
  Gain1 : Gain  Gain=a1
  Gain5 : Gain  Gain=a2
  Sum : Sum  Inputs=|+-
  Sum1 : Sum  Inputs=|+-
  Sum5 : Sum  Inputs=|+-
  Filtered state : Outport
  wires:
  Bus Creator/1 -> Filtered state/1
  Angle/1 -> Sum/1
  Sum/1 -> Sum5/1
  Gain/1 -> Sum/2
  Gain1/1 -> Sum5/2
  Gain3/1 -> Bus Creator/1  "y"
  Gain2/1 -> Bus Creator/3  "y_ddot"
  Gain4/1 -> Bus Creator/2  "y_dot"
  Gain5/1 -> Sum1/2
  Sum5/1 -> Sum1/1
  Sum1/1 -> Discrete-Time Integrator/1
  Discrete-Time Integrator/1 -> Discrete-Time Integrator1/1, Gain2/1, Gain5/1
  Discrete-Time Integrator1/1 -> Discrete-Time Integrator2/1, Gain4/1, Gain1/1
  Discrete-Time Integrator2/1 -> Gain3/1, Gain/1

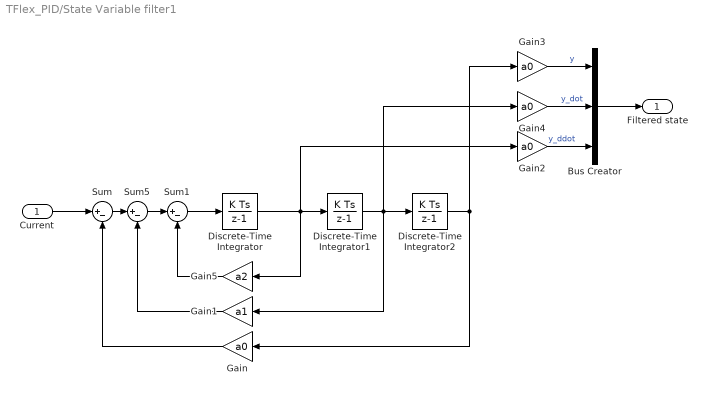
== system TFlex_PID/State Variable filter1 ==
  Current : Inport
  Bus Creator : BusCreator  Inputs=3
  Discrete-Time Integrator : DiscreteIntegrator  SampleTime=-1  ICPrevOutput=DiscIntNeverNeededParam  ICPrevScaledInput=DiscIntNeverNeededParam
  Discrete-Time Integrator1 : DiscreteIntegrator  SampleTime=-1  ICPrevOutput=DiscIntNeverNeededParam  ICPrevScaledInput=DiscIntNeverNeededParam
  Discrete-Time Integrator2 : DiscreteIntegrator  SampleTime=-1  ICPrevOutput=DiscIntNeverNeededParam  ICPrevScaledInput=DiscIntNeverNeededParam
  Gain{,2..4} (4 alike) : Gain  Gain=a0
  Gain1 : Gain  Gain=a1
  Gain5 : Gain  Gain=a2
  Sum : Sum  Inputs=|+-
  Sum1 : Sum  Inputs=|+-
  Sum5 : Sum  Inputs=|+-
  Filtered state : Outport
  wires:
  Bus Creator/1 -> Filtered state/1
  Current/1 -> Sum/1
  Sum/1 -> Sum5/1
  Gain/1 -> Sum/2
  Gain1/1 -> Sum5/2
  Gain3/1 -> Bus Creator/1  "y"
  Gain2/1 -> Bus Creator/3  "y_ddot"
  Gain4/1 -> Bus Creator/2  "y_dot"
  Gain5/1 -> Sum1/2
  Sum5/1 -> Sum1/1
  Sum1/1 -> Discrete-Time Integrator/1
  Discrete-Time Integrator/1 -> Discrete-Time Integrator1/1, Gain2/1, Gain5/1
  Discrete-Time Integrator1/1 -> Discrete-Time Integrator2/1, Gain4/1, Gain1/1
  Discrete-Time Integrator2/1 -> Gain3/1, Gain/1

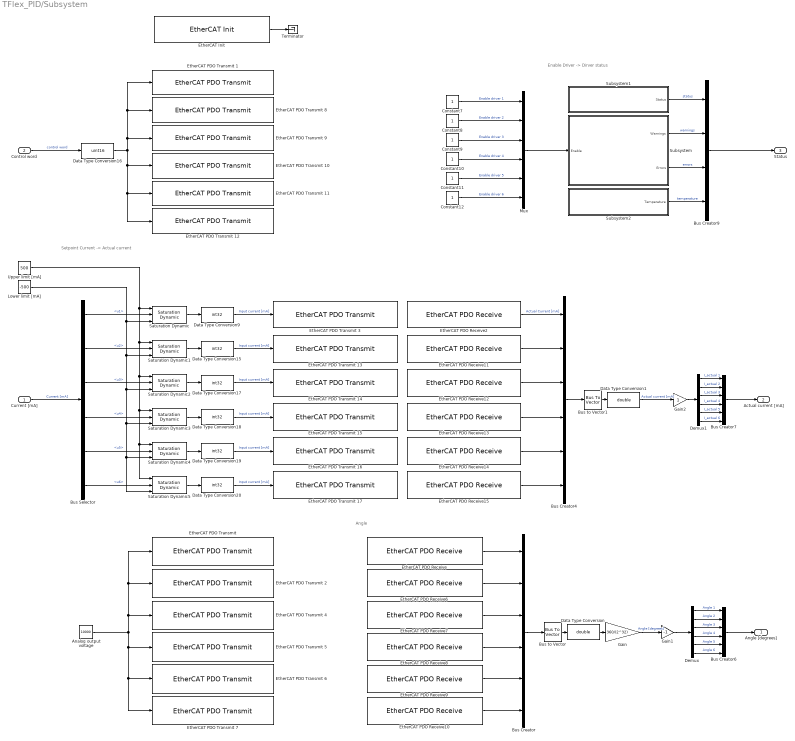
== system TFlex_PID/Subsystem ==
  note: Angle
  note: Enable Driver -> Dirver status
  note: Setpoint Current -> Actual current
  Current [mA] : Inport  PortDimensions=6
  Control word : Inport  Port=2
  Analog output voltage : Constant  Value=10000  OutDataTypeStr=int16  SampleTime=-1
  Bus Creator{,4,6..7} (4 alike) : BusCreator  Inputs=6
  Bus Creator9 : BusCreator  Inputs=4
  Bus Selector : BusSelector  OutputSignals=u1,u2,u3,u4,u5,u6
  Bus to Vector : BusToVector
  Bus to Vector1 : BusToVector
  Constant{7..12} (6 alike) : Constant  OutDataTypeStr=int32  SampleTime=1
  Data Type Conversion : DataTypeConversion  OutDataTypeStr=double
  Data Type Conversion1 : DataTypeConversion  OutDataTypeStr=double
  Data Type Conversion{9,15,17..20} (6 alike) : DataTypeConversion  OutDataTypeStr=int32
  Data Type Conversion16 : DataTypeConversion  OutDataTypeStr=uint16
  Demux : Demux  Outputs=6
  Demux1 : Demux  Outputs=6
  "EtherCAT Init " : xpcethercatlib/EtherCAT Init   Priority=0  config_file=C:\Users\wout7\Documents\GitHub\Inverse_dynamics_learning\TargetPC\6 DOF\pdo_mapping_6dr_1kHz.xml  device_id=0  pci_bus=13  pci_slot=0  pci_function=0  dctuning=0  enaDebug=off  enaDC=on  errLink=off  masterDbg=off  stateChgDbg=off  baseClock=off  masterCfg=off  logFile='c:\dbglog.txt'  sample_time=0.001000  DCMode=2
      settings: SourceProductName=Simulink Real-Time  SourceProductBaseCode=XP
  EtherCAT PDO Receive : xpcethercatlib/EtherCAT PDO Receive  Priority=2  sig_name=Drive 2 (AKD).Inputs_1.Position actual internal value  sig_offset=560  sig_type=int32  type_size=32  sig_dim=1  device_id=0  sample_time=0.001000
      settings: SourceProductName=Simulink Real-Time  SourceProductBaseCode=XP
  EtherCAT PDO Receive10 : xpcethercatlib/EtherCAT PDO Receive  Priority=2  sig_name=Drive 7 (AKD).Inputs_1.Position actual internal value  sig_offset=37488  sig_type=int32  type_size=32  sig_dim=1  device_id=0  sample_time=0.001000
      settings: SourceProductName=Simulink Real-Time  SourceProductBaseCode=XP
  EtherCAT PDO Receive11 : xpcethercatlib/EtherCAT PDO Receive  Priority=2  sig_name=Drive 3 (AKD).Inputs_1.Current actual value  sig_offset=12560  sig_type=int32  type_size=32  sig_dim=1  device_id=0  sample_time=0.001000
      settings: SourceProductName=Simulink Real-Time  SourceProductBaseCode=XP
  EtherCAT PDO Receive12 : xpcethercatlib/EtherCAT PDO Receive  Priority=2  sig_name=Drive 4 (AKD).Inputs_1.Current actual value  sig_offset=24848  sig_type=int32  type_size=32  sig_dim=1  device_id=0  sample_time=0.001000
      settings: SourceProductName=Simulink Real-Time  SourceProductBaseCode=XP
  EtherCAT PDO Receive13 : xpcethercatlib/EtherCAT PDO Receive  Priority=2  sig_name=Drive 5 (AKD).Inputs_1.Current actual value  sig_offset=37136  sig_type=int32  type_size=32  sig_dim=1  device_id=0  sample_time=0.001000
      settings: SourceProductName=Simulink Real-Time  SourceProductBaseCode=XP
  EtherCAT PDO Receive14 : xpcethercatlib/EtherCAT PDO Receive  Priority=2  sig_name=Drive 6 (AKD).Inputs_1.Current actual value  sig_offset=37296  sig_type=int32  type_size=32  sig_dim=1  device_id=0  sample_time=0.001000
      settings: SourceProductName=Simulink Real-Time  SourceProductBaseCode=XP
  EtherCAT PDO Receive15 : xpcethercatlib/EtherCAT PDO Receive  Priority=2  sig_name=Drive 7 (AKD).Inputs_1.Current actual value  sig_offset=37456  sig_type=int32  type_size=32  sig_dim=1  device_id=0  sample_time=0.001000
      settings: SourceProductName=Simulink Real-Time  SourceProductBaseCode=XP
  EtherCAT PDO Receive2 : xpcethercatlib/EtherCAT PDO Receive  Priority=2  sig_name=Drive 2 (AKD).Inputs_1.Current actual value  sig_offset=528  sig_type=int32  type_size=32  sig_dim=1  device_id=0  sample_time=0.001000
      settings: SourceProductName=Simulink Real-Time  SourceProductBaseCode=XP
  EtherCAT PDO Receive6 : xpcethercatlib/EtherCAT PDO Receive  Priority=2  sig_name=Drive 3 (AKD).Inputs_1.Position actual internal value  sig_offset=12592  sig_type=int32  type_size=32  sig_dim=1  device_id=0  sample_time=0.001000
      settings: SourceProductName=Simulink Real-Time  SourceProductBaseCode=XP
  EtherCAT PDO Receive7 : xpcethercatlib/EtherCAT PDO Receive  Priority=2  sig_name=Drive 4 (AKD).Inputs_1.Position actual internal value  sig_offset=24880  sig_type=int32  type_size=32  sig_dim=1  device_id=0  sample_time=0.001000
      settings: SourceProductName=Simulink Real-Time  SourceProductBaseCode=XP
  EtherCAT PDO Receive8 : xpcethercatlib/EtherCAT PDO Receive  Priority=2  sig_name=Drive 5 (AKD).Inputs_1.Position actual internal value  sig_offset=37168  sig_type=int32  type_size=32  sig_dim=1  device_id=0  sample_time=0.001000
      settings: SourceProductName=Simulink Real-Time  SourceProductBaseCode=XP
  EtherCAT PDO Receive9 : xpcethercatlib/EtherCAT PDO Receive  Priority=2  sig_name=Drive 6 (AKD).Inputs_1.Position actual internal value  sig_offset=37328  sig_type=int32  type_size=32  sig_dim=1  device_id=0  sample_time=0.001000
      settings: SourceProductName=Simulink Real-Time  SourceProductBaseCode=XP
  "EtherCAT PDO Transmit " : xpcethercatlib/EtherCAT PDO Transmit   Priority=3  sig_name=Drive 2 (AKD).Outputs.AOUT.VALUE write  sig_offset=480  sig_type=int16  type_size=16  sig_dim=1  device_id=0  sample_time=0.001000
      settings: SourceProductName=Simulink Real-Time  SourceProductBaseCode=XP
  EtherCAT PDO Transmit 1 : xpcethercatlib/EtherCAT PDO Transmit   Priority=3  sig_name=Drive 2 (AKD).Outputs.Controlword  sig_offset=464  sig_type=uint16  type_size=16  sig_dim=1  device_id=0  sample_time=0.001000
      settings: SourceProductName=Simulink Real-Time  SourceProductBaseCode=XP
  EtherCAT PDO Transmit 10 : xpcethercatlib/EtherCAT PDO Transmit   Priority=3  sig_name=Drive 5 (AKD).Outputs.Controlword  sig_offset=37072  sig_type=uint16  type_size=16  sig_dim=1  device_id=0  sample_time=0.001000
      settings: SourceProductName=Simulink Real-Time  SourceProductBaseCode=XP
  EtherCAT PDO Transmit 11 : xpcethercatlib/EtherCAT PDO Transmit   Priority=3  sig_name=Drive 6 (AKD).Outputs.Controlword  sig_offset=37232  sig_type=uint16  type_size=16  sig_dim=1  device_id=0  sample_time=0.001000
      settings: SourceProductName=Simulink Real-Time  SourceProductBaseCode=XP
  EtherCAT PDO Transmit 12 : xpcethercatlib/EtherCAT PDO Transmit   Priority=3  sig_name=Drive 7 (AKD).Outputs.Controlword  sig_offset=37392  sig_type=uint16  type_size=16  sig_dim=1  device_id=0  sample_time=0.001000
      settings: SourceProductName=Simulink Real-Time  SourceProductBaseCode=XP
  EtherCAT PDO Transmit 13 : xpcethercatlib/EtherCAT PDO Transmit   Priority=3  sig_name=Drive 3 (AKD).Outputs.Target current  sig_offset=12528  sig_type=int32  type_size=32  sig_dim=1  device_id=0  sample_time=0.001000
      settings: SourceProductName=Simulink Real-Time  SourceProductBaseCode=XP
  EtherCAT PDO Transmit 14 : xpcethercatlib/EtherCAT PDO Transmit   Priority=3  sig_name=Drive 4 (AKD).Outputs.Target current  sig_offset=24816  sig_type=int32  type_size=32  sig_dim=1  device_id=0  sample_time=0.001000
      settings: SourceProductName=Simulink Real-Time  SourceProductBaseCode=XP
  EtherCAT PDO Transmit 15 : xpcethercatlib/EtherCAT PDO Transmit   Priority=3  sig_name=Drive 5 (AKD).Outputs.Target current  sig_offset=37104  sig_type=int32  type_size=32  sig_dim=1  device_id=0  sample_time=0.001000
      settings: SourceProductName=Simulink Real-Time  SourceProductBaseCode=XP
  EtherCAT PDO Transmit 16 : xpcethercatlib/EtherCAT PDO Transmit   Priority=3  sig_name=Drive 6 (AKD).Outputs.Target current  sig_offset=37264  sig_type=int32  type_size=32  sig_dim=1  device_id=0  sample_time=0.001000
      settings: SourceProductName=Simulink Real-Time  SourceProductBaseCode=XP
  EtherCAT PDO Transmit 17 : xpcethercatlib/EtherCAT PDO Transmit   Priority=3  sig_name=Drive 7 (AKD).Outputs.Target current  sig_offset=37424  sig_type=int32  type_size=32  sig_dim=1  device_id=0  sample_time=0.001000
      settings: SourceProductName=Simulink Real-Time  SourceProductBaseCode=XP
  EtherCAT PDO Transmit 2 : xpcethercatlib/EtherCAT PDO Transmit   Priority=3  sig_name=Drive 3 (AKD).Outputs.AOUT.VALUE write  sig_offset=12512  sig_type=int16  type_size=16  sig_dim=1  device_id=0  sample_time=0.001000
      settings: SourceProductName=Simulink Real-Time  SourceProductBaseCode=XP
  EtherCAT PDO Transmit 3 : xpcethercatlib/EtherCAT PDO Transmit   Priority=3  sig_name=Drive 2 (AKD).Outputs.Target current  sig_offset=496  sig_type=int32  type_size=32  sig_dim=1  device_id=0  sample_time=0.001000
      settings: SourceProductName=Simulink Real-Time  SourceProductBaseCode=XP
  EtherCAT PDO Transmit 4 : xpcethercatlib/EtherCAT PDO Transmit   Priority=3  sig_name=Drive 4 (AKD).Outputs.AOUT.VALUE write  sig_offset=24800  sig_type=int16  type_size=16  sig_dim=1  device_id=0  sample_time=0.001000
      settings: SourceProductName=Simulink Real-Time  SourceProductBaseCode=XP
  EtherCAT PDO Transmit 5 : xpcethercatlib/EtherCAT PDO Transmit   Priority=3  sig_name=Drive 5 (AKD).Outputs.AOUT.VALUE write  sig_offset=37088  sig_type=int16  type_size=16  sig_dim=1  device_id=0  sample_time=0.001000
      settings: SourceProductName=Simulink Real-Time  SourceProductBaseCode=XP
  EtherCAT PDO Transmit 6 : xpcethercatlib/EtherCAT PDO Transmit   Priority=3  sig_name=Drive 6 (AKD).Outputs.AOUT.VALUE write  sig_offset=37248  sig_type=int16  type_size=16  sig_dim=1  device_id=0  sample_time=0.001000
      settings: SourceProductName=Simulink Real-Time  SourceProductBaseCode=XP
  EtherCAT PDO Transmit 7 : xpcethercatlib/EtherCAT PDO Transmit   Priority=3  sig_name=Drive 7 (AKD).Outputs.AOUT.VALUE write  sig_offset=37408  sig_type=int16  type_size=16  sig_dim=1  device_id=0  sample_time=0.001000
      settings: SourceProductName=Simulink Real-Time  SourceProductBaseCode=XP
  EtherCAT PDO Transmit 8 : xpcethercatlib/EtherCAT PDO Transmit   Priority=3  sig_name=Drive 3 (AKD).Outputs.Controlword  sig_offset=12496  sig_type=uint16  type_size=16  sig_dim=1  device_id=0  sample_time=0.001000
      settings: SourceProductName=Simulink Real-Time  SourceProductBaseCode=XP
  EtherCAT PDO Transmit 9 : xpcethercatlib/EtherCAT PDO Transmit   Priority=3  sig_name=Drive 4 (AKD).Outputs.Controlword  sig_offset=24784  sig_type=uint16  type_size=16  sig_dim=1  device_id=0  sample_time=0.001000
      settings: SourceProductName=Simulink Real-Time  SourceProductBaseCode=XP
  Gain : Gain  Gain=360/(2^32)
  Gain1 : Gain  Gain=-1
  Gain2 : Gain
  Lower limit [mA] : Constant  Value=-500  SampleTime=ts
  Mux : Mux  Inputs=6
  Saturation Dynamic{,1..5} (6 alike) : simulink/Discontinuities/Saturation Dynamic  OutMin=[]  OutMax=[]  OutDataTypeStr=Inherit: Same as second input  OutDataType=fixdt(1, 16)  OutScaling=2^-10  DoSatur=off
  Subsystem : Subsystem
  Subsystem1 : Subsystem
  Subsystem2 : Subsystem
  Terminator : Terminator
  Upper limit [mA] : Constant  Value=500  SampleTime=ts
  Angle [degrees] : Outport
  Actual current [mA] : Outport  Port=2
  Status : Outport  Port=3
  wires:
  EtherCAT PDO Receive12/1 -> Bus Creator4/3
  Upper limit [mA]/1 -> Saturation Dynamic3/1, Saturation Dynamic4/1, Saturation Dynamic5/1, Saturation Dynamic2/1, Saturation Dynamic1/1, Saturation Dynamic/1
  Bus Selector/1 -> Saturation Dynamic/2  "<u1>"
  Analog output voltage/1 -> EtherCAT PDO Transmit 7/1, EtherCAT PDO Transmit 6/1, EtherCAT PDO Transmit 5/1, "EtherCAT PDO Transmit "/1, EtherCAT PDO Transmit 2/1, EtherCAT PDO Transmit 4/1
  Bus Selector/4 -> Saturation Dynamic3/2  "<u4>"
  Saturation Dynamic/1 -> Data Type Conversion9/1
  Bus to Vector1/1 -> Data Type Conversion1/1
  EtherCAT PDO Receive2/1 -> Bus Creator4/1  "Actual Current [mA]"
  EtherCAT PDO Receive6/1 -> Bus Creator/2
  Saturation Dynamic5/1 -> Data Type Conversion20/1
  EtherCAT PDO Receive10/1 -> Bus Creator/6
  Data Type Conversion20/1 -> EtherCAT PDO Transmit 17/1  "Input current [mA]"
  Bus Selector/3 -> Saturation Dynamic2/2  "<u3>"
  EtherCAT PDO Receive9/1 -> Bus Creator/5
  Saturation Dynamic4/1 -> Data Type Conversion19/1
  Bus Selector/2 -> Saturation Dynamic1/2  "<u2>"
  EtherCAT PDO Receive7/1 -> Bus Creator/3
  Data Type Conversion/1 -> Gain/1
  Gain/1 -> Gain1/1  "Angle [degrees]"
  Demux/6 -> Bus Creator6/6  "Angle 6"
  Current [mA]/1 -> Bus Selector/1  "Current [mA]"
  Control word/1 -> Data Type Conversion16/1  "control word"
  Demux/3 -> Bus Creator6/3  "Angle 3"
  Bus Creator9/1 -> Status/1
  Saturation Dynamic3/1 -> Data Type Conversion18/1
  Data Type Conversion18/1 -> EtherCAT PDO Transmit 15/1  "Input current [mA]"
  Demux1/3 -> Bus Creator7/3  "I_actual 3"
  Bus Creator4/1 -> Bus to Vector1/1
  Data Type Conversion17/1 -> EtherCAT PDO Transmit 14/1  "Input current [mA]"
  Saturation Dynamic1/1 -> Data Type Conversion15/1
  Demux1/2 -> Bus Creator7/2  "I_actual 2"
  Demux/4 -> Bus Creator6/4  "Angle 4"
  Bus Selector/5 -> Saturation Dynamic4/2  "<u5>"
  Data Type Conversion16/1 -> EtherCAT PDO Transmit 1/1, EtherCAT PDO Transmit 8/1, EtherCAT PDO Transmit 9/1, EtherCAT PDO Transmit 12/1, EtherCAT PDO Transmit 11/1, EtherCAT PDO Transmit 10/1
  EtherCAT PDO Receive/1 -> Bus Creator/1
  EtherCAT PDO Receive15/1 -> Bus Creator4/6
  Data Type Conversion15/1 -> EtherCAT PDO Transmit 13/1  "Input current [mA]"
  Bus to Vector/1 -> Data Type Conversion/1
  Data Type Conversion19/1 -> EtherCAT PDO Transmit 16/1  "Input current [mA]"
  Demux/1 -> Bus Creator6/1  "Angle 1"
  Lower limit [mA]/1 -> Saturation Dynamic/3, Saturation Dynamic1/3, Saturation Dynamic2/3, Saturation Dynamic3/3, Saturation Dynamic4/3, Saturation Dynamic5/3
  EtherCAT PDO Receive13/1 -> Bus Creator4/4
  "EtherCAT Init "/1 -> Terminator/1
  Data Type Conversion1/1 -> Gain2/1  "Actual current [mA]"
  Demux/5 -> Bus Creator6/5  "Angle 5"
  Demux1/4 -> Bus Creator7/4  "I_actual 4"
  Demux1/6 -> Bus Creator7/6  "I_actual 6"
  Bus Creator/1 -> Bus to Vector/1
  EtherCAT PDO Receive11/1 -> Bus Creator4/2
  Bus Selector/6 -> Saturation Dynamic5/2  "<u6>"
  EtherCAT PDO Receive14/1 -> Bus Creator4/5
  Data Type Conversion9/1 -> EtherCAT PDO Transmit 3/1  "Input current [mA]"
  EtherCAT PDO Receive8/1 -> Bus Creator/4
  Demux1/1 -> Bus Creator7/1  "I_actual 1"
  Demux1/5 -> Bus Creator7/5  "I_actual 5"
  Demux/2 -> Bus Creator6/2  "Angle 2"
  Bus Creator6/1 -> Angle [degrees]/1
  Saturation Dynamic2/1 -> Data Type Conversion17/1
  Bus Creator7/1 -> Actual current [mA]/1
  Constant7/1 -> Mux/1  "Enable driver 1"
  Constant8/1 -> Mux/2  "Enable driver 2"
  Constant9/1 -> Mux/3  "Enable driver 3"
  Constant10/1 -> Mux/4  "Enable driver 4"
  Constant11/1 -> Mux/5  "Enable driver 5"
  Constant12/1 -> Mux/6  "Enable driver 6"
  Mux/1 -> Subsystem/1(Enable)
  Subsystem/1(Warnings) -> Bus Creator9/2  "warnings"
  Subsystem/2(Errors) -> Bus Creator9/3  "errors"
  Subsystem1/1(Status) -> Bus Creator9/1  "status"
  Subsystem2/1(Temperature) -> Bus Creator9/4  "temperature"
  Gain1/1 -> Demux/1
  Gain2/1 -> Demux1/1

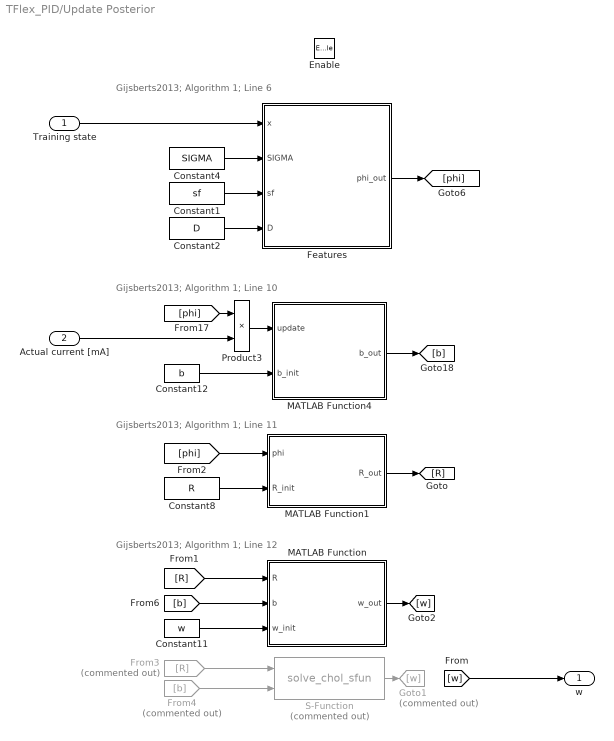
== system TFlex_PID/Update Posterior ==
  note: Gijsberts2013; Algorithm 1; Line 6
  note: Gijsberts2013; Algorithm 1; Line 10
  note: Gijsberts2013; Algorithm 1; Line 11
  note: Gijsberts2013; Algorithm 1; Line 12
  Training state : Inport
  "Actual current [mA] " : Inport  Port=2
  Enable : EnablePort
  Constant1 : Constant  Value=sf  VectorParams1D=off
  Constant11 : Constant  Value=w  VectorParams1D=off  SampleTime=ts
  Constant12 : Constant  Value=b  VectorParams1D=off  SampleTime=ts
  Constant2 : Constant  Value=D  VectorParams1D=off
  Constant4 : Constant  Value=SIGMA  VectorParams1D=off
  Constant8 : Constant  Value=R  VectorParams1D=off  SampleTime=ts
  Features : Subsystem
  From3 : From  Commented=on  GotoTag=R
  From4 : From  Commented=on  GotoTag=b
  Goto1 : Goto  Commented=on  GotoTag=w
  MATLAB Function : MATLAB Function  TreatAsAtomicUnit=on
  MATLAB Function1 : MATLAB Function  TreatAsAtomicUnit=on
  MATLAB Function4 : MATLAB Function  TreatAsAtomicUnit=on
  Product3 : Product
  S-Function : S-Function  Commented=on  FunctionName=solve_chol_sfun  Parameters=2*D  SFunctionDeploymentMode=off  EnableBusSupport=off
  w : Outport
  wires:
  [phi] -> MATLAB Function1/1(phi)
  Training state/1 -> Features/1(x)
  Features/1(phi_out) -> [phi]
  MATLAB Function1/1(R_out) -> [R]
  Constant4/1 -> Features/2(SIGMA)
  [R] -> MATLAB Function/1(R)
  [b] -> MATLAB Function/2(b)
  Constant8/1 -> MATLAB Function1/2(R_init)
  Constant11/1 -> MATLAB Function/3(w_init)
  "Actual current [mA] "/1 -> Product3/2
  [phi] -> Product3/1
  Product3/1 -> MATLAB Function4/1(update)
  Constant12/1 -> MATLAB Function4/2(b_init)
  MATLAB Function4/1(b_out) -> [b]
  S-Function/1 -> Goto1/1
  [w] -> w/1
  From3/1 -> S-Function/1
  From4/1 -> S-Function/2
  MATLAB Function/1(w_out) -> [w]
  Constant1/1 -> Features/3(sf)
  Constant2/1 -> Features/4(D)

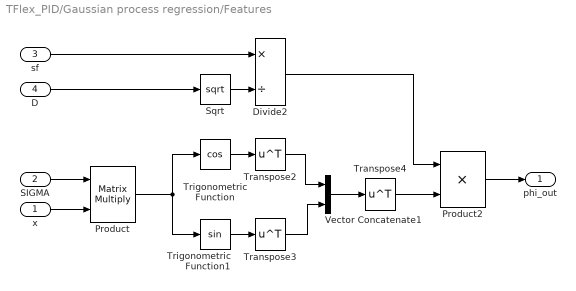
== system TFlex_PID/Gaussian process regression/Features ==
  x : Inport
  SIGMA : Inport  Port=2
  sf : Inport  Port=3
  D : Inport  Port=4
  Divide2 : Product  Inputs=*/
  Product : Product  Multiplication=Matrix(*)
  Product2 : Product
  Sqrt : Sqrt  SaturateOnIntegerOverflow=on
  Transpose2 : Math  Operator=transpose  SaturateOnIntegerOverflow=on
  Transpose3 : Math  Operator=transpose  SaturateOnIntegerOverflow=on
  Transpose4 : Math  Operator=transpose  SaturateOnIntegerOverflow=on
  Trigonometric Function : Trigonometry  Operator=cos
  Trigonometric Function1 : Trigonometry
  Vector Concatenate1 : Concatenate
  phi_out : Outport
  wires:
  SIGMA/1 -> Product/1
  Product2/1 -> phi_out/1
  D/1 -> Sqrt/1
  Trigonometric Function1/1 -> Transpose3/1
  Trigonometric Function/1 -> Transpose2/1
  sf/1 -> Divide2/1
  Vector Concatenate1/1 -> Transpose4/1
  Transpose3/1 -> Vector Concatenate1/2
  Product/1 -> Trigonometric Function1/1, Trigonometric Function/1
  Divide2/1 -> Product2/1
  Transpose4/1 -> Product2/2
  Sqrt/1 -> Divide2/2
  Transpose2/1 -> Vector Concatenate1/1
  x/1 -> Product/2

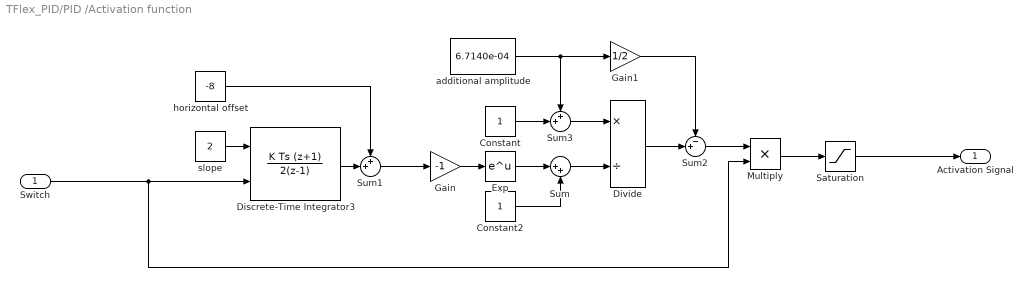
== system TFlex_PID/PID /Activation function ==
  Switch : Inport
  Constant : Constant
  Constant2 : Constant
  Discrete-Time Integrator3 : DiscreteIntegrator  IntegratorMethod=Integration: Trapezoidal  ExternalReset=rising  SampleTime=-1  UpperSaturationLimit=1  LowerSaturationLimit=0  ICPrevOutput=DiscIntNeverNeededParam  ICPrevScaledInput=DiscIntNeverNeededParam
  Divide : Product  Inputs=*/
  Exp : Math  SaturateOnIntegerOverflow=on
  Gain : Gain  Gain=-1
  Gain1 : Gain  Gain=1/2
  Multiply : Product
  Saturation : Saturate  UpperLimit=1  LowerLimit=0
  Sum : Sum  Inputs=|++
  Sum1 : Sum  Inputs=++|
  Sum2 : Sum  Inputs=-+|
  Sum3 : Sum  Inputs=++|
  additional amplitude : Constant  Value=6.7140e-04
  horizontal offset : Constant  Value=-8
  slope : Constant  Value=2
  Activation Signal : Outport
  wires:
  Constant/1 -> Sum3/2
  Exp/1 -> Sum/1
  additional amplitude/1 -> Sum3/1, Gain1/1
  Sum1/1 -> Gain/1
  Gain1/1 -> Sum2/1
  Divide/1 -> Sum2/2
  Sum/1 -> Divide/2
  Gain/1 -> Exp/1
  slope/1 -> Discrete-Time Integrator3/1
  Discrete-Time Integrator3/1 -> Sum1/2
  Constant2/1 -> Sum/2
  Sum2/1 -> Multiply/1
  Sum3/1 -> Divide/1
  horizontal offset/1 -> Sum1/1
  Saturation/1 -> Activation Signal/1
  Multiply/1 -> Saturation/1
  Switch/1 -> Multiply/2, Discrete-Time Integrator3/2
